simulink model "SF103A_MotRefMdl"  (R2013b)
settings: Solver=FixedStepDiscrete  StartTime=0.0  StopTime=2  FixedStep=.002  RelTol=1e-3
values from neighbouring files (symbols this model uses):
  ARCHGLBPRM_2MILLISEC_SEC_F32 = DataDict.Constant    [SF103A_MotRefMdl_DataDict.m]
  ARCHGLBPRM_2OVERSQRT3_ULS_F32 = DataDict.Constant    [SF103A_MotRefMdl_DataDict.m]
  ARCHGLBPRM_2PI_ULS_F32 = DataDict.Constant    [SF103A_MotRefMdl_DataDict.m]
  ARCHGLBPRM_4OVERSQRT3_ULS_F32 = DataDict.Constant    [SF103A_MotRefMdl_DataDict.m]
  ARCHGLBPRM_5PIOVER4_ULS_F32 = DataDict.Constant    [SF103A_MotRefMdl_DataDict.m]
  ARCHGLBPRM_FLOATZEROTHD_ULS_F32 = DataDict.Constant    [SF103A_MotRefMdl_DataDict.m]
  ARCHGLBPRM_HALFSQRT3_ULS_F32 = DataDict.Constant    [SF103A_MotRefMdl_DataDict.m]
  ARCHGLBPRM_PI_ULS_F32 = DataDict.Constant    [SF103A_MotRefMdl_DataDict.m]
  MotRefMdlCurrDaxBoostGain = DataDict.Calibration    [SF103A_MotRefMdl_DataDict.m]
  MotRefMdlCurrDaxQaxRefDelta = DataDict.Calibration    [SF103A_MotRefMdl_DataDict.m]
  MotRefMdlCurrItrnTolr = DataDict.Calibration    [SF103A_MotRefMdl_DataDict.m]
  MotRefMdlFbCtrlDi = DataDict.Calibration    [SF103A_MotRefMdl_DataDict.m]
  MotRefMdlIvtrDeadTiBrdgVltgSca = DataDict.Calibration    [SF103A_MotRefMdl_DataDict.m]
  MotRefMdlMinCurrItrnLim = DataDict.Calibration    [SF103A_MotRefMdl_DataDict.m]
  MotRefMdlMotCurrDaxMaxSca = DataDict.Calibration    [SF103A_MotRefMdl_DataDict.m]
  MotRefMdlMotVltgDerivtvTiCon = DataDict.Calibration    [SF103A_MotRefMdl_DataDict.m]
  MotRefMdlRefLocnItrnLim = DataDict.Calibration    [SF103A_MotRefMdl_DataDict.m]
  MotRefMdlTqItrnLim = DataDict.Calibration    [SF103A_MotRefMdl_DataDict.m]
  MotRefMdlTqItrnTolr = DataDict.Calibration    [SF103A_MotRefMdl_DataDict.m]
  MotRefMdlVltgModDynCmpEna = DataDict.Calibration    [SF103A_MotRefMdl_DataDict.m]
  MotRefMdlVltgOverRThdSca = DataDict.Calibration    [SF103A_MotRefMdl_DataDict.m]
  SysGlbPrmMotPoleCnt = DataDict.ImprtdCal    [SF103A_MotRefMdl_DataDict.m]
undefined symbols (not defined in the file or in its folder): MotQuad1
libraries: NxtrLim x19, simulink x4, LnrIntrpn x3, Fil x2, NxtrAbslt x2, FixdToFloat x2, FloatToFixd x2, NxtrMath x1
(part 3 of 7)

== system SF103A_MotRefMdl/MotRefMdl/MotRefMdlPer1/LocateTorqueExtremes ==
  note: Code is not using upper/mid/lower structure as in model.  It is
      | using EA3-style arrays of [x1, y1, x2, y2, x3, y3].  Needs to be
      | revisited.  Code match model, or model match code?
  note: Search the established Delta brackets for the largest motor torque value of the same sign
      | as the Motor Torque Command and output the index value of that maximum
  note: Compute the corresponding Iq and Id values at each of the 8 delta angles
  note: Determine the maximum possible motor torque and the corresponding direct axis current that corresponds to that torque at the present
      | operating point by using the Intermediate calculation terms and the sign of the torque command.  In order to do this, a series of search
      |  brackets are created by rotating the voltage vector completely around a circle in a finite number of steps. Then the bracket array is
      | searched for the maximum torque. If the resulting brackets include an angle of zero, the brackets are adjusted to wrap the angle and
      | avoid a discontinuity at zero. Finally, iterative parabolic interpolation is used to refine the location of the maximum torque.
  note: Calculate Torque
  note: -------------------------- Choose Delta Brackets ------------------------------
  note: VSinCosToIdIq
  note: Find Peak Torques
  note: NOTE:
      | Zero-based indexing
  note: These blocks intenionally placed outside iterator.
  MotTqCmd : Inport  RequirementInfo={} %GIDa_d67c909c_7802_4dca_8c4a_b8b8931c6374
  InterCalcns : Inport  RequirementInfo={} %GIDa_8380d7a7_c13f_42e8_98d3_dcc3fffc1a1a  Port=2
  Add : Sum  RequirementInfo={'linktype_rmi_doors' '0000bb42 (/E-STEER Core/SubSystem Specifications/Application Functions/SF99/SF103A Motor Reference Model)' '#SF103A_94' 'true' 'REQ:SF103A_94' '' } %GIDa_9920bf3e_5a95_4f31_9590_3ee92424380d
  Bus Selector1 : BusSelector  RequirementInfo={'linktype_rmi_doors' '0000bb42 (/E-STEER Core/SubSystem Specifications/Application Functions/SF99/SF103A Motor Reference Model)' '#SF103A_94' 'true' 'REQ:SF103A_94' '' } %GIDa_28e0e43d_816c_4930_83ca_80d107317549  OutputSignals=ReacncDaxOverR,VovrRovrZ_Ampr,EgOverROverZ_Ampr,ReacncQaxOverR,VltgOverR_Ampr
  CalculateTorque : Subsystem  RequirementInfo={'linktype_rmi_doors' '0000bb42 (/E-STEER Core/SubSystem Specifications/Application Functions/SF99/SF103A Motor Reference Model)' '#SF103A_95' 'true' 'REQ:SF103A_95' '' } %GIDa_2397f9a3_9d9c_4815_af52_108914571b1f  TreatAsAtomicUnit=on
  CopyRight2 : Subsystem  Description=|  mask(Copyright Information){none=on}
      | Copyright info block.                                               
      |                                                                     
      | Place copyright information at the top of every subsystem in design.
      mask prompts: none "No parameters"
      mask help: Place copyright information at the top of every subsystem in design.
      mask Display:
      | NxtrConf = 'Nexteer Confidential';
      | 
      | sys = bdroot; %handle for the current model ("system")
      | first = get_param(sys,'Created');
      | first = first(end-3:end);  %year is last four digits
      | 
      | last = get_param(sys,'LastModifiedDate');
      | if isempty(last)
      |     last = datestr(now,'yyyy');
      | else
      |     last = last(end-3:end);
      | end
      | 
      | if strcmp(first,last)
      |     fprintf('%s -- Copyright %s Nexteer',NxtrConf,first)
      | else
      |     fprintf('%s -- %s%s- %s Nexteer',NxtrConf,char(169),first,last)
      | end
  Data Store Read : DataStoreRead  DataStoreName=CosDelta
  Data Store Read1 : DataStoreRead  DataStoreName=SinDelta
  DisplayVar1 : DataStoreWrite  DataStoreName=dMotRefMdlPeakTqNrItrn
  DisplayVar2 : DataStoreWrite  DataStoreName=dMotRefMdlPhaAdvAtPeakTq
  DisplayVar3 : DataStoreWrite  DataStoreName=dMotRefMdlCurrDaxAtPeakTq
  DisplayVar4 : DataStoreWrite  DataStoreName=dMotRefMdlPeakTq
  If : If  RequirementInfo={'linktype_rmi_doors' '0000bb42 (/E-STEER Core/SubSystem Specifications/Application Functions/SF99/SF103A Motor Reference Model)' '#SF103A_97' 'true' 'REQ:SF103A_97' '' } %GIDa_9e36a805_816c_4407_8349_abf5a1df7080  IfExpression=u1 >= 0
  InterpolatePeakTorque : Subsystem  RequirementInfo={'linktype_rmi_doors' '0000bb42 (/E-STEER Core/SubSystem Specifications/Application Functions/SF99/SF103A Motor Reference Model)' '#SF103A_138' 'true' 'REQ:SF103A_138' '' ; 'linktype_rmi_doors' '0000bb42 (/E-STEER Core/SubSystem Specifications/Application Functions/SF99/SF103A Motor Reference Model)' '#SF103A_101' 'true' 'REQ:SF103A_101' '' } %GIDa_8a0f4e37_e388_4d93_8f33_3b322c76185d  TreatAsAtomicUnit=on
  Merge : Merge  RequirementInfo={'linktype_rmi_doors' '0000bb42 (/E-STEER Core/SubSystem Specifications/Application Functions/SF99/SF103A Motor Reference Model)' '#SF103A_97' 'true' 'REQ:SF103A_97' '' } %GIDa_3ac7f0ac_18f8_48ab_a150_8cf50c466b94
  Negative : Subsystem  RequirementInfo={'linktype_rmi_doors' '0000bb42 (/E-STEER Core/SubSystem Specifications/Application Functions/SF99/SF103A Motor Reference Model)' '#SF103A_97' 'true' 'REQ:SF103A_97' '' } %GIDa_6b946297_1610_4b9f_9aff_e8a8f06a5f5a  TreatAsAtomicUnit=on
      settings: RTWSystemCode=Inline
  Positive : Subsystem  RequirementInfo={'linktype_rmi_doors' '0000bb42 (/E-STEER Core/SubSystem Specifications/Application Functions/SF99/SF103A Motor Reference Model)' '#SF103A_97' 'true' 'REQ:SF103A_97' '' } %GIDa_91b2437d_9546_419b_9079_f7367649d9ad  TreatAsAtomicUnit=on
      settings: RTWSystemCode=Inline
  Product : Product  RequirementInfo={'linktype_rmi_doors' '0000bb42 (/E-STEER Core/SubSystem Specifications/Application Functions/SF99/SF103A Motor Reference Model)' '#SF103A_94' 'true' 'REQ:SF103A_94' '' } %GIDa_309b0c3c_bd7c_43e6_9cc7_22b194f1380d
  Product1 : Product  RequirementInfo={'linktype_rmi_doors' '0000bb42 (/E-STEER Core/SubSystem Specifications/Application Functions/SF99/SF103A Motor Reference Model)' '#SF103A_94' 'true' 'REQ:SF103A_94' '' } %GIDa_bae8a1dd_22ed_4dae_b6b5_f5b7807c2904
  Product2 : Product  RequirementInfo={'linktype_rmi_doors' '0000bb42 (/E-STEER Core/SubSystem Specifications/Application Functions/SF99/SF103A Motor Reference Model)' '#SF103A_94' 'true' 'REQ:SF103A_94' '' } %GIDa_2d5ee5d8_1b0c_4b41_ac87_34901100fa76
  Product3 : Product  RequirementInfo={'linktype_rmi_doors' '0000bb42 (/E-STEER Core/SubSystem Specifications/Application Functions/SF99/SF103A Motor Reference Model)' '#SF103A_94' 'true' 'REQ:SF103A_94' '' } %GIDa_1be17003_54b5_407b_a208_77e7f2b83335
  Subtract : Sum  RequirementInfo={'linktype_rmi_doors' '0000bb42 (/E-STEER Core/SubSystem Specifications/Application Functions/SF99/SF103A Motor Reference Model)' '#SF103A_94' 'true' 'REQ:SF103A_94' '' } %GIDa_f5db4b1a_d174_4488_8076_9ec420d2ef61  Inputs=+-
  Subtract1 : Sum  RequirementInfo={'linktype_rmi_doors' '0000bb42 (/E-STEER Core/SubSystem Specifications/Application Functions/SF99/SF103A Motor Reference Model)' '#SF103A_94' 'true' 'REQ:SF103A_94' '' } %GIDa_d1acb025_6416_4554_b7d2_635602019607  Inputs=+-
  WrapBracketAngles : Subsystem  RequirementInfo={'linktype_rmi_doors' '0000bb42 (/E-STEER Core/SubSystem Specifications/Application Functions/SF99/SF103A Motor Reference Model)' '#SF103A_138' 'true' 'REQ:SF103A_138' '' ; 'linktype_rmi_doors' '0000bb42 (/E-STEER Core/SubSystem Specifications/Application Functions/SF99/SF103A Motor Reference Model)' '#SF103A_100' 'true' 'REQ:SF103A_100' '' } %GIDa_f1cafe9a_d050_4041_bb9d_53a0cd4a5df8
  PeakTq : Outport
  CurrDaxAtPeakTq : Outport  Port=2
  wires:
  InterCalcns/1 -> InterpolatePeakTorque/2(InterCalcns), CalculateTorque/3(In2), Bus Selector1/1
  Bus Selector1/1 -> Product/2  "<ReacncDaxOverR>"
  Add/1 -> Product1/1
  Bus Selector1/2 -> Product1/2  "<VovrRovrZ_Ampr>"
  Product1/1 -> Subtract/1
  Bus Selector1/3 -> Subtract/2  "<EgOverROverZ_Ampr>"
  Subtract/1 -> Product2/1, CalculateTorque/2(CurrQax)  "CurrQax_Amp"
  Bus Selector1/4 -> Product2/2  "<ReacncQaxOverR>"
  Bus Selector1/5 -> Product3/1  "<VltgOverR_Ampr>"
  Data Store Read1/1 -> Product/1, Product3/2
  Product/1 -> Add/2
  Product2/1 -> Subtract1/1
  Product3/1 -> Subtract1/2
  WrapBracketAngles/1(IntrpnPts) -> InterpolatePeakTorque/1(IntrpnPts)
  MotTqCmd/1 -> If/1
  If/1 -> Positive/Action
  If/2 -> Negative/Action
  Positive/1(IdxSt) -> Merge/1
  Negative/1(IdxSt) -> Merge/2
  Merge/1 -> WrapBracketAngles/2(IdxSt)  "IdxSt"
  CalculateTorque/1(TqAry) -> Negative/1(TqAry), Positive/1(TqAry), WrapBracketAngles/1(TqAry)
  Subtract1/1 -> CalculateTorque/1(CurrDax)  "CurrDax_Amp"
  InterpolatePeakTorque/2(Delta) -> DisplayVar2/1
  InterpolatePeakTorque/1(NrItrn) -> DisplayVar1/1
  InterpolatePeakTorque/3(CurrDaxRef) -> DisplayVar3/1, CurrDaxAtPeakTq/1
  InterpolatePeakTorque/4(Tq) -> DisplayVar4/1, PeakTq/1
  Data Store Read/1 -> Add/1

== system SF103A_MotRefMdl/MotRefMdl/MotRefMdlPer1/MotCurrAg_AlphaCalc ==
  note: The Motor Reference Current Angle Calculation performs an ATAN2 calculation on the
      | Motor Reference Current - D Axis and Motor Reference Current Q - Axis for use by
      | the Current Measurement function.
  note: /* Motor CurrentAngle Computation */
  MotCurrDaxCmd : Inport  RequirementInfo={} %GIDa_69639cde_f2be_4855_b9da_73ff0545938e
  MotCurrQaxCmd : Inport  RequirementInfo={} %GIDa_fc08e164_b6ec_4351_a17e_4cefb6448169  Port=2
  CopyRight2 : Subsystem  Description=|  mask(Copyright Information){none=on}
      | Copyright info block.                                               
      |                                                                     
      | Place copyright information at the top of every subsystem in design.
      mask prompts: none "No parameters"
      mask help: Place copyright information at the top of every subsystem in design.
      mask Display:
      | NxtrConf = 'Nexteer Confidential';
      | 
      | sys = bdroot; %handle for the current model ("system")
      | first = get_param(sys,'Created');
      | first = first(end-3:end);  %year is last four digits
      | 
      | last = get_param(sys,'LastModifiedDate');
      | if isempty(last)
      |     last = datestr(now,'yyyy');
      | else
      |     last = last(end-3:end);
      | end
      | 
      | if strcmp(first,last)
      |     fprintf('%s -- Copyright %s Nexteer',NxtrConf,first)
      | else
      |     fprintf('%s -- %s%s- %s Nexteer',NxtrConf,char(169),first,last)
      | end
  If : If  IfExpression=u1 < 0
  Merge : Merge
  No Wrapping : Subsystem  TreatAsAtomicUnit=on
      settings: AttributesFormatString=pass_thru
  Wrap Angle : Subsystem  TreatAsAtomicUnit=on
  atan2 : Trigonometry  RequirementInfo={'linktype_rmi_doors' '0000bb42 (/E-STEER Core/SubSystem Specifications/Application Functions/SF99/SF103A Motor Reference Model)' '#SF103A_131' 'true' 'REQ:SF103A_131' '' } %GIDa_7d407f85_e635_488f_93ef_72a7530532e1  Operator=atan2
  MotCurrAg_Rad : Outport  RequirementInfo={} %GIDa_1b268fe2_8de8_4dfd_94c4_6b9021bf2617
  wires:
  MotCurrQaxCmd/1 -> atan2/2
  MotCurrDaxCmd/1 -> atan2/1
  If/1 -> Wrap Angle/Action
  If/2 -> No Wrapping/Action
  atan2/1 -> No Wrapping/1(In1), Wrap Angle/1(In1), If/1
  Wrap Angle/1(Out1) -> Merge/1
  No Wrapping/1(Out1) -> Merge/2
  Merge/1 -> MotCurrAg_Rad/1

== system SF103A_MotRefMdl/MotRefMdl/MotRefMdlPer1/VoltageScheduling ==
  note: The Voltage Scheduling subfunction calculates and applies a gain scaling and an offset value
      |  to the measured DC Link voltage.The adjusted voltage value (Voltage Supply Available) is used
      |  as the constraint supply voltage in the subsequent reference current calculations.
  MotVelFild : Inport  RequirementInfo={} %GIDa_b1302cbd_1280_4e9c_ba99_35fce541a303
  MotQuad : Inport  RequirementInfo={} %GIDa_c9b7cebe_749c_4e3f_b79f_e2207d300931  Port=2
  BrdgVltgLimd : Inport  RequirementInfo={} %GIDa_a03bfab4_537e_4a55_83a8_e7ece775eb88  Port=3
  Abslt_f32_f32 : NxtrAbslt/Abslt_f32_f32  RequirementInfo={'linktype_rmi_doors' '0000bb42 (/E-STEER Core/SubSystem Specifications/Application Functions/SF99/SF103A Motor Reference Model)' '#SF103A_75' 'true' 'REQ:SF103A_75' '' ; 'linktype_rmi_doors' '0000bb42 (/E-STEER Core/SubSystem Specifications/Application Functions/SF99/SF103A Motor Reference Model)' '#SF103A_76' 'true' 'REQ:SF103A_76' '' } %GIDa_26e4854a_e21e_4ab6_a271_fd7236401934  SFunctionSpec=single y1 = Abslt_f32_f32(single u1)
      settings: AttributesFormatString=%<Name>
  Constant : Constant  RequirementInfo={'linktype_rmi_doors' '0000bb42 (/E-STEER Core/SubSystem Specifications/Application Functions/SF99/SF103A Motor Reference Model)' '#SF103A_74' 'true' 'REQ:SF103A_74' '' } %GIDa_ef45d06e_31be_46c1_859e_ea7cc2cd22ab  Value=MotRefMdlIvtrDeadTiBrdgVltgSca
  CopyRight2 : Subsystem  Description=|  mask(Copyright Information){none=on}
      | Copyright info block.                                               
      |                                                                     
      | Place copyright information at the top of every subsystem in design.
      mask prompts: none "No parameters"
      mask help: Place copyright information at the top of every subsystem in design.
      mask Display:
      | NxtrConf = 'Nexteer Confidential';
      | 
      | sys = bdroot; %handle for the current model ("system")
      | first = get_param(sys,'Created');
      | first = first(end-3:end);  %year is last four digits
      | 
      | last = get_param(sys,'LastModifiedDate');
      | if isempty(last)
      |     last = datestr(now,'yyyy');
      | else
      |     last = last(end-3:end);
      | end
      | 
      | if strcmp(first,last)
      |     fprintf('%s -- Copyright %s Nexteer',NxtrConf,first)
      | else
      |     fprintf('%s -- %s%s- %s Nexteer',NxtrConf,char(169),first,last)
      | end
  Enumerated_Constant : simulink/Sources/Enumerated Constant  RequirementInfo={'linktype_rmi_doors' '0000bb42 (/E-STEER Core/SubSystem Specifications/Application Functions/SF99/SF103A Motor Reference Model)' '#SF103A_75' 'true' 'REQ:SF103A_75' '' ; 'linktype_rmi_doors' '0000bb42 (/E-STEER Core/SubSystem Specifications/Application Functions/SF99/SF103A Motor Reference Model)' '#SF103A_76' 'true' 'REQ:SF103A_76' '' ; 'linktype_rmi_doors' '0000bb42 (/E-STEER Core/SubSystem Specifications/Application Functions/SF99/SF103A Motor Reference Model)' '#SF103A_77' 'true' 'REQ:SF103A_77' '' ; 'linktype_rmi_doors' '0000bb42 (/E-STEER Core/SubSystem Specifications/Application Functions/SF99/SF103A Motor Reference Model)' '#SF103A_178' 'true' 'REQ:SF103A_178' '' } %GIDa_65f250d7_dd15_4c2a_a627_daefb3e5dadd  OutDataTypeStr=Enum: MotQuad1  Value=MotQuad1.MOTQUAD_QUAD3  SampleTime=inf
  Enumerated_Constant2 : simulink/Sources/Enumerated Constant  RequirementInfo={'linktype_rmi_doors' '0000bb42 (/E-STEER Core/SubSystem Specifications/Application Functions/SF99/SF103A Motor Reference Model)' '#SF103A_75' 'true' 'REQ:SF103A_75' '' ; 'linktype_rmi_doors' '0000bb42 (/E-STEER Core/SubSystem Specifications/Application Functions/SF99/SF103A Motor Reference Model)' '#SF103A_76' 'true' 'REQ:SF103A_76' '' ; 'linktype_rmi_doors' '0000bb42 (/E-STEER Core/SubSystem Specifications/Application Functions/SF99/SF103A Motor Reference Model)' '#SF103A_77' 'true' 'REQ:SF103A_77' '' ; 'linktype_rmi_doors' '0000bb42 (/E-STEER Core/SubSystem Specifications/Application Functions/SF99/SF103A Motor Reference Model)' '#SF103A_178' 'true' 'REQ:SF103A_178' '' } %GIDa_14c3b1f8_2572_48ce_96bd_133f5857719f  OutDataTypeStr=Enum: MotQuad1  Value=MotQuad1.MOTQUAD_QUAD1  SampleTime=inf
  FixdToFloat_f32_u16 : FixdToFloat/FixdToFloat_f32_u16  RequirementInfo={'linktype_rmi_doors' '0000bb42 (/E-STEER Core/SubSystem Specifications/Application Functions/SF99/SF103A Motor Reference Model)' '#SF103A_76' 'true' 'REQ:SF103A_76' '' } %GIDa_21002382_75bd_4df9_89a7_76b9e6d71e46  Param1=13
  FloatToFixd_u16_f32 : FloatToFixd/FloatToFixd_u16_f32  RequirementInfo={'linktype_rmi_doors' '0000bb42 (/E-STEER Core/SubSystem Specifications/Application Functions/SF99/SF103A Motor Reference Model)' '#SF103A_75' 'true' 'REQ:SF103A_75' '' } %GIDa_db5708a1_cc71_4c3b_ab3b_49bc3c499ce9  Param1=5
  If : If  RequirementInfo={'linktype_rmi_doors' '0000bb42 (/E-STEER Core/SubSystem Specifications/Application Functions/SF99/SF103A Motor Reference Model)' '#SF103A_75' 'true' 'REQ:SF103A_75' '' ; 'linktype_rmi_doors' '0000bb42 (/E-STEER Core/SubSystem Specifications/Application Functions/SF99/SF103A Motor Reference Model)' '#SF103A_76' 'true' 'REQ:SF103A_76' '' ; 'linktype_rmi_doors' '0000bb42 (/E-STEER Core/SubSystem Specifications/Application Functions/SF99/SF103A Motor Reference Model)' '#SF103A_77' 'true' 'REQ:SF103A_77' '' ; 'linktype_rmi_doors' '0000bb42 (/E-STEER Core/SubSystem Specifications/Application Functions/SF99/SF103A Motor Reference Model)' '#SF103A_178' 'true' 'REQ:SF103A_178' '' } %GIDa_d41c1b26_0037_467b_b116_dc4db21cbfbf  NumInputs=2  IfExpression=u1 | u2
  If Action Subsystem : Subsystem  RequirementInfo={'linktype_rmi_doors' '0000bb42 (/E-STEER Core/SubSystem Specifications/Application Functions/SF99/SF103A Motor Reference Model)' '#SF103A_75' 'true' 'REQ:SF103A_75' '' ; 'linktype_rmi_doors' '0000bb42 (/E-STEER Core/SubSystem Specifications/Application Functions/SF99/SF103A Motor Reference Model)' '#SF103A_76' 'true' 'REQ:SF103A_76' '' ; 'linktype_rmi_doors' '0000bb42 (/E-STEER Core/SubSystem Specifications/Application Functions/SF99/SF103A Motor Reference Model)' '#SF103A_77' 'true' 'REQ:SF103A_77' '' ; 'linktype_rmi_doors' '0000bb42 (/E-STEER Core/SubSystem Specifications/Application Functions/SF99/SF103A Motor Reference Model)' '#SF103A_178' 'true' 'REQ:SF103A_178' '' } %GIDa_3864d4de_0cb1_404c_9515_20e72fd37b55  TreatAsAtomicUnit=on
      settings: RTWSystemCode=Inline
  If Action Subsystem1 : Subsystem  RequirementInfo={'linktype_rmi_doors' '0000bb42 (/E-STEER Core/SubSystem Specifications/Application Functions/SF99/SF103A Motor Reference Model)' '#SF103A_75' 'true' 'REQ:SF103A_75' '' ; 'linktype_rmi_doors' '0000bb42 (/E-STEER Core/SubSystem Specifications/Application Functions/SF99/SF103A Motor Reference Model)' '#SF103A_76' 'true' 'REQ:SF103A_76' '' ; 'linktype_rmi_doors' '0000bb42 (/E-STEER Core/SubSystem Specifications/Application Functions/SF99/SF103A Motor Reference Model)' '#SF103A_77' 'true' 'REQ:SF103A_77' '' ; 'linktype_rmi_doors' '0000bb42 (/E-STEER Core/SubSystem Specifications/Application Functions/SF99/SF103A Motor Reference Model)' '#SF103A_178' 'true' 'REQ:SF103A_178' '' } %GIDa_43384ae2_1e49_4f72_aee7_641de4786986  TreatAsAtomicUnit=on
      settings: RTWSystemCode=Inline
  LimStat_f32 : NxtrLim/LimStat_f32  RequirementInfo={'linktype_rmi_doors' '0000bb42 (/E-STEER Core/SubSystem Specifications/Application Functions/SF99/SF103A Motor Reference Model)' '#SF103A_74' 'true' 'REQ:SF103A_74' '' } %GIDa_45b86618_03f3_4afa_9b83_c66df7651775  LoLim=MOTREFMDL_INVTERDEADTIBRDGVLTGSCALOLIM_ULS_F32  HiLim=MOTREFMDL_INVTERDEADTIBRDGVLTGSCAHILIM_ULS_F32
      settings: AttributesFormatString=|
      | Low Limit: %<LoLim>
      | High Limit:%<HiLim>
  Merge : Merge  RequirementInfo={'linktype_rmi_doors' '0000bb42 (/E-STEER Core/SubSystem Specifications/Application Functions/SF99/SF103A Motor Reference Model)' '#SF103A_75' 'true' 'REQ:SF103A_75' '' ; 'linktype_rmi_doors' '0000bb42 (/E-STEER Core/SubSystem Specifications/Application Functions/SF99/SF103A Motor Reference Model)' '#SF103A_76' 'true' 'REQ:SF103A_76' '' ; 'linktype_rmi_doors' '0000bb42 (/E-STEER Core/SubSystem Specifications/Application Functions/SF99/SF103A Motor Reference Model)' '#SF103A_77' 'true' 'REQ:SF103A_77' '' ; 'linktype_rmi_doors' '0000bb42 (/E-STEER Core/SubSystem Specifications/Application Functions/SF99/SF103A Motor Reference Model)' '#SF103A_178' 'true' 'REQ:SF103A_178' '' } %GIDa_f312a83d_8f86_4e06_8e90_0ebc8f6b9c19
  Product : Product  RequirementInfo={'linktype_rmi_doors' '0000bb42 (/E-STEER Core/SubSystem Specifications/Application Functions/SF99/SF103A Motor Reference Model)' '#SF103A_74' 'true' 'REQ:SF103A_74' '' } %GIDa_3f622dbd_19ab_415c_b947_7f5c24dfebaa  RndMeth=Zero
  Relational Operator : RelationalOperator  RequirementInfo={'linktype_rmi_doors' '0000bb42 (/E-STEER Core/SubSystem Specifications/Application Functions/SF99/SF103A Motor Reference Model)' '#SF103A_75' 'true' 'REQ:SF103A_75' '' ; 'linktype_rmi_doors' '0000bb42 (/E-STEER Core/SubSystem Specifications/Application Functions/SF99/SF103A Motor Reference Model)' '#SF103A_76' 'true' 'REQ:SF103A_76' '' ; 'linktype_rmi_doors' '0000bb42 (/E-STEER Core/SubSystem Specifications/Application Functions/SF99/SF103A Motor Reference Model)' '#SF103A_77' 'true' 'REQ:SF103A_77' '' ; 'linktype_rmi_doors' '0000bb42 (/E-STEER Core/SubSystem Specifications/Application Functions/SF99/SF103A Motor Reference Model)' '#SF103A_178' 'true' 'REQ:SF103A_178' '' } %GIDa_ec09dbf9_2859_4cdc_be21_f5c25f498aa5  Operator===  OutDataTypeStr=boolean
  Relational Operator1 : RelationalOperator  RequirementInfo={'linktype_rmi_doors' '0000bb42 (/E-STEER Core/SubSystem Specifications/Application Functions/SF99/SF103A Motor Reference Model)' '#SF103A_75' 'true' 'REQ:SF103A_75' '' ; 'linktype_rmi_doors' '0000bb42 (/E-STEER Core/SubSystem Specifications/Application Functions/SF99/SF103A Motor Reference Model)' '#SF103A_76' 'true' 'REQ:SF103A_76' '' ; 'linktype_rmi_doors' '0000bb42 (/E-STEER Core/SubSystem Specifications/Application Functions/SF99/SF103A Motor Reference Model)' '#SF103A_77' 'true' 'REQ:SF103A_77' '' ; 'linktype_rmi_doors' '0000bb42 (/E-STEER Core/SubSystem Specifications/Application Functions/SF99/SF103A Motor Reference Model)' '#SF103A_178' 'true' 'REQ:SF103A_178' '' } %GIDa_7cda9388_137e_478f_a070_a50998abdc1e  Operator===  OutDataTypeStr=boolean
  Subtract : Sum  RequirementInfo={'linktype_rmi_doors' '0000bb42 (/E-STEER Core/SubSystem Specifications/Application Functions/SF99/SF103A Motor Reference Model)' '#SF103A_78' 'true' 'REQ:SF103A_78' '' } %GIDa_46291f81_ace0_4614_8000_6d2a5faf21e2  Inputs=+-
  VltgSplyAvail : Outport  RequirementInfo={} %GIDa_ace5953b_26aa_4e1f_8585_c9315db42bde
  wires:
  Constant/1 -> LimStat_f32/1
  LimStat_f32/1 -> Product/2
  BrdgVltgLimd/1 -> Product/1
  Product/1 -> Subtract/1
  Subtract/1 -> VltgSplyAvail/1
  Enumerated_Constant2/1 -> Relational Operator/2
  MotQuad/1 -> Relational Operator1/1, Relational Operator/1
  Enumerated_Constant/1 -> Relational Operator1/2
  Relational Operator/1 -> If/1
  Relational Operator1/1 -> If/2
  MotVelFild/1 -> Abslt_f32_f32/1
  If/1 -> If Action Subsystem/Action
  If/2 -> If Action Subsystem1/Action
  Abslt_f32_f32/1 -> FloatToFixd_u16_f32/1
  [Vel] -> If Action Subsystem1/1(AbsMotVelFild)
  [Vel] -> If Action Subsystem/1(AbsMotVelFild)
  If Action Subsystem/1(VltgSdl) -> Merge/1
  If Action Subsystem1/1(VltgSdl) -> Merge/2
  Merge/1 -> FixdToFloat_f32_u16/1
  FloatToFixd_u16_f32/1 -> [Vel]
  FixdToFloat_f32_u16/1 -> Subtract/2

== system SF103A_MotRefMdl/MotRefMdl/MotRefMdlPer1/ApplyTorqueLimit/CopyRight2 ==

== system SF103A_MotRefMdl/MotRefMdl/MotRefMdlPer1/ApplyTorqueLimit/If Action Subsystem ==
  In1 : Inport
  Action Port : ActionPort  ActionType=then
  Out1 : Outport
  wires:
  In1/1 -> Out1/1

== system SF103A_MotRefMdl/MotRefMdl/MotRefMdlPer1/ApplyTorqueLimit/If Action Subsystem1 ==
  In1 : Inport
  Action Port : ActionPort  ActionType=else
  Out1 : Outport
  wires:
  In1/1 -> Out1/1

== system SF103A_MotRefMdl/MotRefMdl/MotRefMdlPer1/CalcMinimumMotorCurrent/CopyRight2 ==

== system SF103A_MotRefMdl/MotRefMdl/MotRefMdlPer1/CalcMinimumMotorCurrent/F_CalcIqCmd_1 ==
  note: Code uses a local function to sum the squares
  IterCalcns : Inport  RequirementInfo={} %GIDa_caf5c323_8139_4cbc_a36d_f3c19fce14b5
  MotTqCmd : Inport  RequirementInfo={} %GIDa_d087170c_d5b8_448e_8348_c75f1c7141e2  Port=2
  "CurrDaxRef " : Inport  RequirementInfo={} %GIDa_b98469bd_0919_423c_b222_0008d58b2b6f  Port=3
  Add : Sum  RequirementInfo={'linktype_rmi_doors' '0000bb42 (/E-STEER Core/SubSystem Specifications/Application Functions/SF99/SF103A Motor Reference Model)' '#SF103A_106' 'true' 'REQ:SF103A_106' '' } %GIDa_1c27e68e_50b8_4ad4_b5b4_f76c68954adc
  Add1 : Sum  RequirementInfo={'linktype_rmi_doors' '0000bb42 (/E-STEER Core/SubSystem Specifications/Application Functions/SF99/SF103A Motor Reference Model)' '#SF103A_107' 'true' 'REQ:SF103A_107' '' } %GIDa_0086b8e5_4002_4848_86e1_37b6a9da7b4e
  Bus Selector : BusSelector  RequirementInfo={} %GIDa_d8315c72_974e_438a_a534_4f06c949ae8c  OutputSignals=Ke_VoltPerRadPerSec,RelncTqCoeff_Henry_f32
  Math Function : Math  RequirementInfo={'linktype_rmi_doors' '0000bb42 (/E-STEER Core/SubSystem Specifications/Application Functions/SF99/SF103A Motor Reference Model)' '#SF103A_107' 'true' 'REQ:SF103A_107' '' } %GIDa_ba90d27c_ec80_4405_b27f_a29f69e716d8  Operator=square  SaturateOnIntegerOverflow=on
  Math Function1 : Math  RequirementInfo={'linktype_rmi_doors' '0000bb42 (/E-STEER Core/SubSystem Specifications/Application Functions/SF99/SF103A Motor Reference Model)' '#SF103A_107' 'true' 'REQ:SF103A_107' '' } %GIDa_1bf6c6e2_712a_490b_93f2_9138f4d1e7b3  Operator=square  SaturateOnIntegerOverflow=on
  Product : Product  RequirementInfo={'linktype_rmi_doors' '0000bb42 (/E-STEER Core/SubSystem Specifications/Application Functions/SF99/SF103A Motor Reference Model)' '#SF103A_106' 'true' 'REQ:SF103A_106' '' } %GIDa_dcb0d6f0_093c_429d_9df8_0176d529b16e  RndMeth=Zero
  Product1 : Product  RequirementInfo={'linktype_rmi_doors' '0000bb42 (/E-STEER Core/SubSystem Specifications/Application Functions/SF99/SF103A Motor Reference Model)' '#SF103A_106' 'true' 'REQ:SF103A_106' '' } %GIDa_fcfc152f_233c_46c0_97b7_e0d749465cf2  Inputs=*/  RndMeth=Zero
  CurrDaxRefUppr : Outport
  CurrQaxRefUppr : Outport  RequirementInfo={} %GIDa_97db39b4_7cc7_48e5_a0a6_8ccf8f94ec82  Port=2
  CurrMagSqRefUppr : Outport  RequirementInfo={} %GIDa_89e0c81e_be08_4cc9_b8d4_3115547f834d  Port=3
  wires:
  MotTqCmd/1 -> Product1/1
  Add/1 -> Product1/2
  Product/1 -> Add/2
  Bus Selector/1 -> Add/1  "<Ke_VoltPerRadPerSec>"
  Bus Selector/2 -> Product/1  "<RelncTqCoeff_Henry_f32>"
  IterCalcns/1 -> Bus Selector/1
  "CurrDaxRef "/1 -> Math Function1/1, CurrDaxRefUppr/1, Product/2  "UpprDelta"
  Product1/1 -> Math Function/1, CurrQaxRefUppr/1  "CurrQaxRefUppr"
  Math Function/1 -> Add1/1
  Add1/1 -> CurrMagSqRefUppr/1  "UpprTq"
  Math Function1/1 -> Add1/2

== system SF103A_MotRefMdl/MotRefMdl/MotRefMdlPer1/CalcMinimumMotorCurrent/F_CalcIqCmd_2 ==
  note: Code uses a local function to sum the squares
  IterCalcns : Inport  RequirementInfo={} %GIDa_96c9e1aa_8e9b_4ccf_8f3f_bf3fecef39b2
  MotTqCmd : Inport  RequirementInfo={} %GIDa_f3e8a9b1_6984_4c1f_8ab3_f7f50e4ae0e9  Port=2
  "CurrDaxRef " : Inport  RequirementInfo={} %GIDa_cfed116e_e933_40e9_a6ba_a79e25846971  Port=3
  Add : Sum  RequirementInfo={'linktype_rmi_doors' '0000bb42 (/E-STEER Core/SubSystem Specifications/Application Functions/SF99/SF103A Motor Reference Model)' '#SF103A_106' 'true' 'REQ:SF103A_106' '' } %GIDa_fb9984aa_4e97_4ee6_af1f_5d3a2886bcb6
  Add1 : Sum  RequirementInfo={'linktype_rmi_doors' '0000bb42 (/E-STEER Core/SubSystem Specifications/Application Functions/SF99/SF103A Motor Reference Model)' '#SF103A_107' 'true' 'REQ:SF103A_107' '' } %GIDa_6a3cc569_892f_47f4_aa5a_5222573452a3
  Bus Selector1 : BusSelector  RequirementInfo={} %GIDa_b224975d_1c76_4317_8fa0_67e3959aa356  OutputSignals=Ke_VoltPerRadPerSec,RelncTqCoeff_Henry_f32
  CopyRight2 : Subsystem  Description=|  mask(Copyright Information){none=on}
      | Copyright info block.                                               
      |                                                                     
      | Place copyright information at the top of every subsystem in design.
      mask prompts: none "No parameters"
      mask help: Place copyright information at the top of every subsystem in design.
      mask Display:
      | NxtrConf = 'Nexteer Confidential';
      | 
      | sys = bdroot; %handle for the current model ("system")
      | first = get_param(sys,'Created');
      | first = first(end-3:end);  %year is last four digits
      | 
      | last = get_param(sys,'LastModifiedDate');
      | if isempty(last)
      |     last = datestr(now,'yyyy');
      | else
      |     last = last(end-3:end);
      | end
      | 
      | if strcmp(first,last)
      |     fprintf('%s -- Copyright %s Nexteer',NxtrConf,first)
      | else
      |     fprintf('%s -- %s%s- %s Nexteer',NxtrConf,char(169),first,last)
      | end
  Math Function : Math  RequirementInfo={'linktype_rmi_doors' '0000bb42 (/E-STEER Core/SubSystem Specifications/Application Functions/SF99/SF103A Motor Reference Model)' '#SF103A_107' 'true' 'REQ:SF103A_107' '' } %GIDa_74895212_87ad_453c_9156_526074c29b64  Operator=square  SaturateOnIntegerOverflow=on
  Math Function1 : Math  RequirementInfo={'linktype_rmi_doors' '0000bb42 (/E-STEER Core/SubSystem Specifications/Application Functions/SF99/SF103A Motor Reference Model)' '#SF103A_107' 'true' 'REQ:SF103A_107' '' } %GIDa_e69e7cf9_3c07_46eb_b326_6522356e441a  Operator=square  SaturateOnIntegerOverflow=on
  Product2 : Product  RequirementInfo={'linktype_rmi_doors' '0000bb42 (/E-STEER Core/SubSystem Specifications/Application Functions/SF99/SF103A Motor Reference Model)' '#SF103A_106' 'true' 'REQ:SF103A_106' '' } %GIDa_74bd40c0_8f4e_44f4_a072_9e30a84e963f  RndMeth=Zero
  Product3 : Product  RequirementInfo={'linktype_rmi_doors' '0000bb42 (/E-STEER Core/SubSystem Specifications/Application Functions/SF99/SF103A Motor Reference Model)' '#SF103A_106' 'true' 'REQ:SF103A_106' '' } %GIDa_f5b3dd60_9cbe_48d7_8669_7b91d791458c  Inputs=*/  RndMeth=Zero
  CurrDaxRefMid : Outport
  CurrMagSqRefMid : Outport  RequirementInfo={} %GIDa_96797754_13b4_43c0_a140_91aaa4a46a1f  Port=2
  wires:
  Add/1 -> Product3/2
  Product2/1 -> Add/2
  Bus Selector1/1 -> Add/1  "<Ke_VoltPerRadPerSec>"
  Bus Selector1/2 -> Product2/1  "<RelncTqCoeff_Henry_f32>"
  IterCalcns/1 -> Bus Selector1/1
  MotTqCmd/1 -> Product3/1
  "CurrDaxRef "/1 -> Math Function1/1, CurrDaxRefMid/1, Product2/2  "MidDelta"
  Product3/1 -> Math Function/1  "CurrQaxRefMid"
  Math Function/1 -> Add1/1
  Add1/1 -> CurrMagSqRefMid/1  "MidTq"
  Math Function1/1 -> Add1/2

== system SF103A_MotRefMdl/MotRefMdl/MotRefMdlPer1/CalcMinimumMotorCurrent/If Action Subsystem ==
  In1 : Inport
  In2 : Inport  Port=2
  Action Port : ActionPort  ActionType=else
  Out1 : Outport
  Out2 : Outport  Port=2
  wires:
  In1/1 -> Out1/1
  In2/1 -> Out2/1

== system SF103A_MotRefMdl/MotRefMdl/MotRefMdlPer1/CalcMinimumMotorCurrent/If Action Subsystem1 ==
  In1 : Inport
  In2 : Inport  Port=2
  Action Port : ActionPort  ActionType=then
  Out1 : Outport
  Out2 : Outport  Port=2
  wires:
  In1/1 -> Out1/1
  In2/1 -> Out2/1

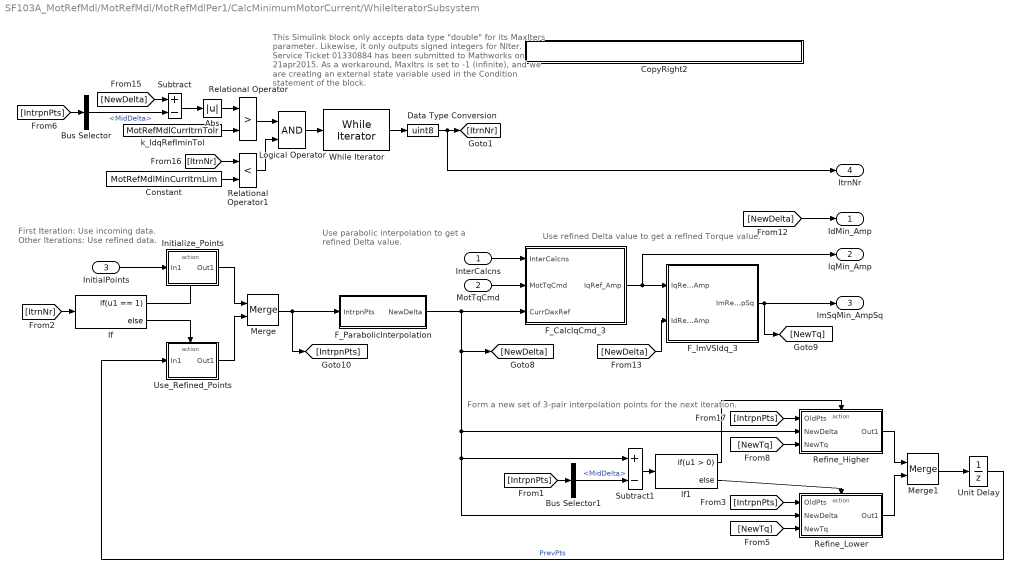
== system SF103A_MotRefMdl/MotRefMdl/MotRefMdlPer1/CalcMinimumMotorCurrent/WhileIteratorSubsystem ==
  note: Form a new set of 3-pair interpolation points for the next iteration.
  note: Use refined Delta value to get a refined Torque value.
  note: Use parabolic interpolation to get
      | a refined Delta value.
  note: First Iteration:      Use incoming data.
      | Other Iterations:  Use refined data.
  note: This Simulink block only accepts data type "double" for its MaxIters parameter.
      | Likewise, it only outputs signed integers for NIter.
      | Service Ticket 01330884 has been submitted to Mathworks on 21apr2015.
      |
      | As a workaround, MaxItrs is set to -1 (infinite), and we are creating an external
      | state variable used in the Condition statement of the block.
  InterCalcns : Inport  RequirementInfo={} %GIDa_77550f74_1515_4e8c_8cf4_af6ae631f2a3
  MotTqCmd : Inport  RequirementInfo={} %GIDa_8c9ee9da_ee0b_44de_92d3_eec01063a537  Port=2
  InitialPoints : Inport  RequirementInfo={} %GIDa_2ea65474_82fc_4dda_9ef6_e6939d050862  Port=3
  Abs : Abs  RequirementInfo={'linktype_rmi_doors' '0000bb42 (/E-STEER Core/SubSystem Specifications/Application Functions/SF99/SF103A Motor Reference Model)' '#SF103A_108' 'true' 'REQ:SF103A_108' '' } %GIDa_1f2e0b2d_83d8_4ff9_8c2f_97535bd85d81
  Bus Selector : BusSelector  RequirementInfo={} %GIDa_0228e942_93b9_4563_af62_3ecb947a8cd2  OutputSignals=MidDelta
  Bus Selector1 : BusSelector  RequirementInfo={} %GIDa_93eac060_65c0_432c_bb7d_b2809624471c  OutputSignals=MidDelta
  Constant : Constant  RequirementInfo={'linktype_rmi_doors' '0000bb42 (/E-STEER Core/SubSystem Specifications/Application Functions/SF99/SF103A Motor Reference Model)' '#SF103A_108' 'true' 'REQ:SF103A_108' '' } %GIDa_f5595666_ef60_41a8_bad1_9363d469354f  Value=MotRefMdlMinCurrItrnLim
  CopyRight2 : Subsystem  Description=|  mask(Copyright Information){none=on}
      | Copyright info block.                                               
      |                                                                     
      | Place copyright information at the top of every subsystem in design.
      mask prompts: none "No parameters"
      mask help: Place copyright information at the top of every subsystem in design.
      mask Display:
      | NxtrConf = 'Nexteer Confidential';
      | 
      | sys = bdroot; %handle for the current model ("system")
      | first = get_param(sys,'Created');
      | first = first(end-3:end);  %year is last four digits
      | 
      | last = get_param(sys,'LastModifiedDate');
      | if isempty(last)
      |     last = datestr(now,'yyyy');
      | else
      |     last = last(end-3:end);
      | end
      | 
      | if strcmp(first,last)
      |     fprintf('%s -- Copyright %s Nexteer',NxtrConf,first)
      | else
      |     fprintf('%s -- %s%s- %s Nexteer',NxtrConf,char(169),first,last)
      | end
  Data Type Conversion : DataTypeConversion  RequirementInfo={'linktype_rmi_doors' '0000bb42 (/E-STEER Core/SubSystem Specifications/Application Functions/SF99/SF103A Motor Reference Model)' '#SF103A_108' 'true' 'REQ:SF103A_108' '' } %GIDa_64f2b3b6_4744_4320_913c_da7c0e0e2c73  OutDataTypeStr=uint8
  F_CalcIqCmd_3 : Subsystem  RequirementInfo={'linktype_rmi_doors' '0000bb42 (/E-STEER Core/SubSystem Specifications/Application Functions/SF99/SF103A Motor Reference Model)' '#SF103A_108' 'true' 'REQ:SF103A_108' '' } %GIDa_a4992f05_568d_453b_b3dd_d2ec2cf8251b
  F_ImVSIdq_3 : Subsystem  RequirementInfo={'linktype_rmi_doors' '0000bb42 (/E-STEER Core/SubSystem Specifications/Application Functions/SF99/SF103A Motor Reference Model)' '#SF103A_108' 'true' 'REQ:SF103A_108' '' } %GIDa_380c1fc5_63f1_4515_a048_d16956cb4262  TreatAsAtomicUnit=on
  F_ParabolicInterpolation : Subsystem  RequirementInfo={'linktype_rmi_doors' '0000bb42 (/E-STEER Core/SubSystem Specifications/Application Functions/SF99/SF103A Motor Reference Model)' '#SF103A_108' 'true' 'REQ:SF103A_108' '' } %GIDa_a8b025fe_4c14_469c_bddf_d428680223aa
  If : If  RequirementInfo={'linktype_rmi_doors' '0000bb42 (/E-STEER Core/SubSystem Specifications/Application Functions/SF99/SF103A Motor Reference Model)' '#SF103A_108' 'true' 'REQ:SF103A_108' '' } %GIDa_6f6bfb0f_4188_44a1_ab05_7779a47dfe87  IfExpression=u1 == 1
  If1 : If  RequirementInfo={'linktype_rmi_doors' '0000bb42 (/E-STEER Core/SubSystem Specifications/Application Functions/SF99/SF103A Motor Reference Model)' '#SF103A_108' 'true' 'REQ:SF103A_108' '' } %GIDa_2182ff1f_73ce_4b08_8796_3c9406cb2515
  Initialize_Points : Subsystem  RequirementInfo={'linktype_rmi_doors' '0000bb42 (/E-STEER Core/SubSystem Specifications/Application Functions/SF99/SF103A Motor Reference Model)' '#SF103A_108' 'true' 'REQ:SF103A_108' '' } %GIDa_e71a4ded_b7c5_4c14_a37d_0ab1042e4591  TreatAsAtomicUnit=on
  Logical Operator : Logic  RequirementInfo={'linktype_rmi_doors' '0000bb42 (/E-STEER Core/SubSystem Specifications/Application Functions/SF99/SF103A Motor Reference Model)' '#SF103A_108' 'true' 'REQ:SF103A_108' '' } %GIDa_bc5b8a0c_d024_4ad7_99ba_98b15da01d80  AllPortsSameDT=off  OutDataTypeStr=boolean
  Merge : Merge  RequirementInfo={'linktype_rmi_doors' '0000bb42 (/E-STEER Core/SubSystem Specifications/Application Functions/SF99/SF103A Motor Reference Model)' '#SF103A_108' 'true' 'REQ:SF103A_108' '' } %GIDa_37e4e086_49b1_4d16_b43a_9c9bf5801362
  Merge1 : Merge  RequirementInfo={'linktype_rmi_doors' '0000bb42 (/E-STEER Core/SubSystem Specifications/Application Functions/SF99/SF103A Motor Reference Model)' '#SF103A_108' 'true' 'REQ:SF103A_108' '' } %GIDa_cf7087a0_8dd5_4fdf_938e_74c7082cc3a3
  Refine_Higher : Subsystem  RequirementInfo={'linktype_rmi_doors' '0000bb42 (/E-STEER Core/SubSystem Specifications/Application Functions/SF99/SF103A Motor Reference Model)' '#SF103A_108' 'true' 'REQ:SF103A_108' '' } %GIDa_efa23b8a_1eef_4b47_aa0b_90a49d2e536d  TreatAsAtomicUnit=on
  Refine_Lower : Subsystem  RequirementInfo={'linktype_rmi_doors' '0000bb42 (/E-STEER Core/SubSystem Specifications/Application Functions/SF99/SF103A Motor Reference Model)' '#SF103A_108' 'true' 'REQ:SF103A_108' '' } %GIDa_93ef0a66_d012_424e_aebf_938a41b17678  TreatAsAtomicUnit=on
  Relational Operator : RelationalOperator  RequirementInfo={'linktype_rmi_doors' '0000bb42 (/E-STEER Core/SubSystem Specifications/Application Functions/SF99/SF103A Motor Reference Model)' '#SF103A_108' 'true' 'REQ:SF103A_108' '' } %GIDa_978906d7_f1d5_4d79_81da_2e382405724c  Operator=>  OutDataTypeStr=boolean
  Relational Operator1 : RelationalOperator  RequirementInfo={'linktype_rmi_doors' '0000bb42 (/E-STEER Core/SubSystem Specifications/Application Functions/SF99/SF103A Motor Reference Model)' '#SF103A_108' 'true' 'REQ:SF103A_108' '' } %GIDa_b9ee3d8a_8099_477e_ab21_cd1adf98f664  Operator=<  OutDataTypeStr=boolean
  Subtract : Sum  RequirementInfo={'linktype_rmi_doors' '0000bb42 (/E-STEER Core/SubSystem Specifications/Application Functions/SF99/SF103A Motor Reference Model)' '#SF103A_108' 'true' 'REQ:SF103A_108' '' } %GIDa_fec8c86e_8cf6_47f1_96aa_ef8487f44fd7  Inputs=+-
  Subtract1 : Sum  RequirementInfo={'linktype_rmi_doors' '0000bb42 (/E-STEER Core/SubSystem Specifications/Application Functions/SF99/SF103A Motor Reference Model)' '#SF103A_108' 'true' 'REQ:SF103A_108' '' } %GIDa_32d66e57_ba25_49c6_b6e5_3649079537a2  Inputs=+-
  Unit Delay : UnitDelay  RequirementInfo={'linktype_rmi_doors' '0000bb42 (/E-STEER Core/SubSystem Specifications/Application Functions/SF99/SF103A Motor Reference Model)' '#SF103A_108' 'true' 'REQ:SF103A_108' '' } %GIDa_c5a1cfda_1a41_44c4_b921_fc8a3f129d68  SampleTime=-1
      settings: AttributesFormatString=|
      | Temp Variable
      | No PIM
  Use_Refined_Points : Subsystem  RequirementInfo={'linktype_rmi_doors' '0000bb42 (/E-STEER Core/SubSystem Specifications/Application Functions/SF99/SF103A Motor Reference Model)' '#SF103A_108' 'true' 'REQ:SF103A_108' '' } %GIDa_c86f88e8_bb99_4169_9387_84796316c6ef  TreatAsAtomicUnit=on
  While Iterator : WhileIterator  RequirementInfo={'linktype_rmi_doors' '0000bb42 (/E-STEER Core/SubSystem Specifications/Application Functions/SF99/SF103A Motor Reference Model)' '#SF103A_108' 'true' 'REQ:SF103A_108' '' } %GIDa_38928def_b148_4e9c_af88_828ce8f5d085  MaxIters=-1  WhileBlockType=do-while  ShowIterationPort=on  OutputDataType=int8
      settings: AttributesFormatString=%<MaxIters>
  k_IdqRefIminTol : Constant  RequirementInfo={'linktype_rmi_doors' '0000bb42 (/E-STEER Core/SubSystem Specifications/Application Functions/SF99/SF103A Motor Reference Model)' '#SF103A_108' 'true' 'REQ:SF103A_108' '' } %GIDa_01772efd_2105_4abf_bedb_d5f633887f27  Value=MotRefMdlCurrItrnTolr
  IdMin_Amp : Outport  RequirementInfo={} %GIDa_ff16974b_ab5e_432e_b2cc_88aef5ed661d
  IqMin_Amp : Outport  RequirementInfo={} %GIDa_e80c47ce_802d_4b46_b45e_2c3aeadd447f  Port=2
  ImSqMin_AmpSq : Outport  RequirementInfo={} %GIDa_7942bd28_586c_4018_913a_c98018c12425  Port=3
  ItrnNr : Outport  RequirementInfo={} %GIDa_c8e52e82_ef5d_475e_8a00_8ff9625bf882  Port=4
  wires:
  F_ImVSIdq_3/1(ImRefSq_AmpSq) -> ImSqMin_AmpSq/1, [NewTq]
  F_CalcIqCmd_3/1(IqRef_Amp) -> F_ImVSIdq_3/1(IqRef_Amp), IqMin_Amp/1
  MotTqCmd/1 -> F_CalcIqCmd_3/2(MotTqCmd)
  InterCalcns/1 -> F_CalcIqCmd_3/1(InterCalcns)
  While Iterator/1 -> Data Type Conversion/1
  Merge1/1 -> Unit Delay/1
  Subtract/1 -> Abs/1
  Relational Operator/1 -> Logical Operator/1
  [NewDelta] -> Subtract/1
  [ItrnNr] -> Relational Operator1/1
  Constant/1 -> Relational Operator1/2
  Logical Operator/1 -> While Iterator/1
  Relational Operator1/1 -> Logical Operator/2
  [IntrpnPts] -> Bus Selector/1
  Bus Selector/1 -> Subtract/2  "<MidDelta>"
  InitialPoints/1 -> Initialize_Points/1(In1)
  [ItrnNr] -> If/1
  If1/1 -> Refine_Higher/Action
  If1/2 -> Refine_Lower/Action
  Refine_Higher/1(Out1) -> Merge1/1
  Refine_Lower/1(Out1) -> Merge1/2
  [IntrpnPts] -> Refine_Higher/1(OldPts)
  [IntrpnPts] -> Refine_Lower/1(OldPts)
  [NewTq] -> Refine_Higher/3(NewTq)
  Merge/1 -> [IntrpnPts], F_ParabolicInterpolation/1(IntrpnPts)
  [IntrpnPts] -> Bus Selector1/1
  Unit Delay/1 -> Use_Refined_Points/1(In1)  "PrevPts"
  Subtract1/1 -> If1/1
  [NewTq] -> Refine_Lower/3(NewTq)
  If/1 -> Initialize_Points/Action
  If/2 -> Use_Refined_Points/Action
  Initialize_Points/1(Out1) -> Merge/1
  Use_Refined_Points/1(Out1) -> Merge/2
  Data Type Conversion/1 -> ItrnNr/1, [ItrnNr]
  Abs/1 -> Relational Operator/1
  k_IdqRefIminTol/1 -> Relational Operator/2
  [NewDelta] -> IdMin_Amp/1
  [NewDelta] -> F_ImVSIdq_3/2(IdRef_Amp)
  F_ParabolicInterpolation/1(NewDelta) -> F_CalcIqCmd_3/3("CurrDaxRef "), [NewDelta], Refine_Higher/2(NewDelta), Subtract1/1, Refine_Lower/2(NewDelta)
  Bus Selector1/1 -> Subtract1/2  "<MidDelta>"

== system SF103A_MotRefMdl/MotRefMdl/MotRefMdlPer1/DAxisCurrentBoost/CopyRight2 ==
